simulink model "RollReducedModel_Generated"  (R2023b)
settings: Solver=FixedStepAuto  StartTime=0.0  StopTime=10.0  FixedStep=0.005  RelTol=1e-3
PreLoadFcn:
  | JointParameters
values from neighbouring files (symbols this model uses):
  B_l = 0.5    [JointParameters.m]    (also in MyDict.sldd = 0.5
                
                    
                  )
  B_u = 0.5    [JointParameters.m]    (also in MyDict.sldd = 0.5
                
                    
                  )
  FilterCoeffN = 10    [JointParameters.m]    (also in MyDict.sldd = 10.0
                
                    
                 )
  g = 9.81    [JointParameters.m]    (also in MyDict.sldd = 9.81
                
                    
                 )
  ixposkd = 0    [JointParameters.m]    (also in MyDict.sldd = 0.0
                
                    
                  )
  ixposki = 1    [JointParameters.m]    (also in MyDict.sldd = 1.0
                
                    
                  )
  ixposkp = 12    [JointParameters.m]    (also in MyDict.sldd = 12.0
                
                    
                 )
  ixvelkd = 0    [JointParameters.m]    (also in MyDict.sldd = 0.0
                
                    
                  )
  ixvelki = 5    [JointParameters.m]    (also in MyDict.sldd = 5.0
                
                    
                  )
  ixvelkp = 30    [JointParameters.m]    (also in MyDict.sldd = 30.0
                
                    
                 )
  iyposkd = 0    [JointParameters.m]    (also in MyDict.sldd = 0.0
                
                    
                  )
  iyposki = 1    [JointParameters.m]    (also in MyDict.sldd = 1.0
                
                    
                  )
  iyposkp = 10    [JointParameters.m]    (also in MyDict.sldd = 10.0
                
                    
                 )
  iyvelkd = 0    [JointParameters.m]    (also in MyDict.sldd = 0.0
                
                    
                  )
  iyvelki = 5    [JointParameters.m]    (also in MyDict.sldd = 5.0
                
                    
                  )
  iyvelkp = 20    [JointParameters.m]    (also in MyDict.sldd = 20.0
                
                    
                 )
  J_l = 0.071440709    [JointParameters.m]    (also in MyDict.sldd = 0.071440709
                
                    
          )
  J_u = 0.049103    [JointParameters.m]    (also in MyDict.sldd = 0.049103
                
                    
             )
  JointX_InitialPositionCondition = 0.27    [JointParameters.m]    (also in MyDict.sldd = 0.27
                
                    
                 )
  JointY_InitialPositionCondition = -0.33    [JointParameters.m]    (also in MyDict.sldd = -0.33
                
                    
                )
  L_cg_l = 0.102366    [JointParameters.m]    (also in MyDict.sldd = 0.102366
                
                    
             )
  L_cg_u = 0.066301    [JointParameters.m]    (also in MyDict.sldd = 0.066301
                
                    
             )
  L_l = 0.223793    [JointParameters.m]    (also in MyDict.sldd = 0.223793
                
                    
             )
  L_u = 0.227293    [JointParameters.m]    (also in MyDict.sldd = 0.227293
                
                    
             )
  mass_l = 2.495    [JointParameters.m]    (also in MyDict.sldd = 2.495
                
                    
                )
  mass_u = 2.024    [JointParameters.m]    (also in MyDict.sldd = 2.024
                
                    
                )
  PitchLowerLimit = -0.37    [JointParameters.m]    (also in MyDict.sldd = -0.37
                
                    
                )
  PitchUpperLimit = 0.27    [JointParameters.m]    (also in MyDict.sldd = 0.27
                
                    
                 )
  PitchXMotorSaturation = 50    [JointParameters.m]    (also in MyDict.sldd = 50.0
                
                    
                 )
  PitchXStartThrust = 50    [JointParameters.m]    (also in MyDict.sldd = 50.0
                
                    
                 )
  RollLowerLimit = -0.33    [JointParameters.m]    (also in MyDict.sldd = -0.33
                
                    
                )
  RollUpperLimit = 0.4    [JointParameters.m]    (also in MyDict.sldd = 0.4
                
                    
                  )
  RollYMotorSaturation = 30    [JointParameters.m]    (also in MyDict.sldd = 30.0
                
                    
                 )
  RollYStartThrust = 40    [JointParameters.m]    (also in MyDict.sldd = 40.0
                
                    
                 )
undefined symbols (not defined in the file or in its folder): DiscIntNeverNeededParam
libraries: slpidlib x4
settings Model: DataDictionary=MyDict.sldd  Creator=user  LastModifiedBy=user
settings SolverCC: AlgebraicLoopSolver=TrustRegion
settings OptimizationCC: DefaultParameterBehavior=Inlined  EnhancedBackFolding=on  PassReuseOutputArgsAs=Individual arguments  ZeroExternalMemoryAtStartup=off  ZeroInternalMemoryAtStartup=off  OptimizeBlockOrder=speed  DifferentSizesBufferReuse=on  OptimizationCustomize=off  EfficientTunableParamExpr=on
settings DebuggingCC: ParameterTunabilityLossMsg=error
settings SFSimCC: MATLABDynamicMemAlloc=off
settings RTWCC: Description=Embedded Coder  SystemTargetFile=ert.tlc  GenCodeOnly=on  TemplateMakefile=ert_default_tmf  GenerateReport=on  LaunchReport=on  DataTypeReplacement=CDataTypesFixedWidth  GenerateWebview=on  GenerateCodeMetricsReport=on
settings CodeAppCC: GenerateComments=off  IgnoreCustomStorageClasses=off  OperatorAnnotations=on  SimulinkDataObjDesc=on  SFDataObjDesc=on  SimulinkBlockComments=off
settings ERTTargetCC: TargetLangStandard=C99 (ISO)  GenerateSampleERTMain=on  SupportAbsoluteTime=off  SupportNonFinite=off  SupportComplex=off  InlinedParameterPlacement=NonHierarchical  ERTCustomFileTemplate=example_file_process.tlc  GlobalDataDefinition=InSourceFile  GlobalDataReference=InSourceFile  ERTFilePackagingFormat=Compact  MaxIdInt64=INT64_MAX  MinIdInt64=INT64_MIN  MaxIdUint64=UINT64_MAX  MaxIdInt32=INT32_MAX  MinIdInt32=INT32_MIN  MaxIdUint32=UINT32_MAX  MaxIdInt16=INT16_MAX  MinIdInt16=INT16_MIN  MaxIdUint16=UINT16_MAX  MaxIdInt8=INT8_MAX  MinIdInt8=INT8_MIN  MaxIdUint8=UINT8_MAX

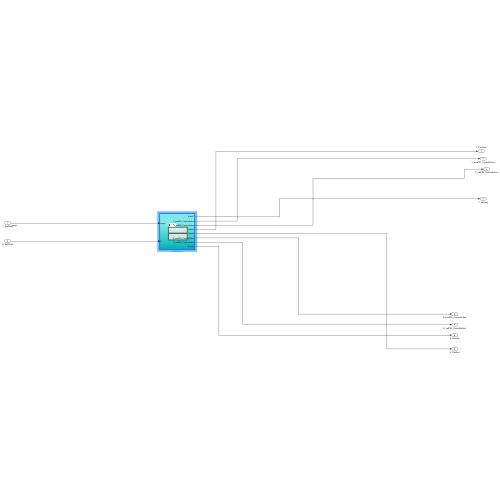
[thumbnail: Simulink's stored preview of the top-level diagram]
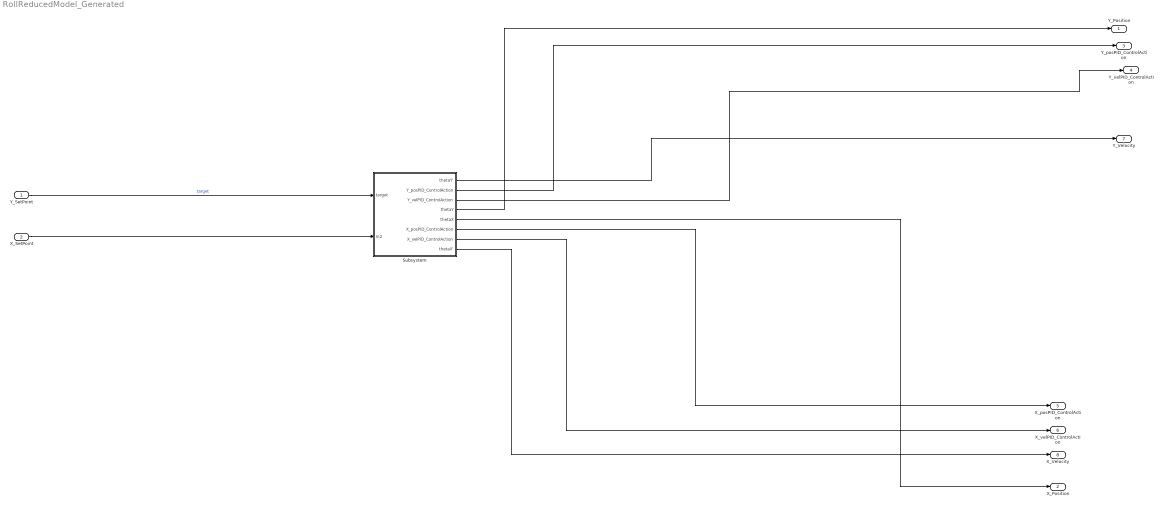
== system RollReducedModel_Generated ==
  Y_SetPoint : Inport  OutDataTypeStr=double
  X_SetPoint : Inport  Port=2  OutDataTypeStr=double
  Subsystem : Subsystem  TreatAsAtomicUnit=on
  Y_Position : Outport
  X_Position : Outport  Port=2
  Y_posPID_ControlAction : Outport  Port=3
  Y_velPID_ControlAction : Outport  Port=4
  X_posPID_ControlAction : Outport  Port=5
  X_velPID_ControlAction : Outport  Port=6
  Y_Velocity : Outport  Port=7
  X_Velocity : Outport  Port=8
  wires:
  Y_SetPoint/1 -> Subsystem/1(target)  "target"
  X_SetPoint/1 -> Subsystem/2(In2)
  Subsystem/1(thetaY') -> Y_Velocity/1
  Subsystem/2(Y_posPID_ControlAction) -> Y_posPID_ControlAction/1
  Subsystem/3(Y_velPID_ControlAction) -> Y_velPID_ControlAction/1
  Subsystem/4(thetaY) -> Y_Position/1
  Subsystem/5(thetaX) -> X_Position/1
  Subsystem/6(X_posPID_ControlAction) -> X_posPID_ControlAction/1
  Subsystem/7(X_velPID_ControlAction) -> X_velPID_ControlAction/1
  Subsystem/8(thetaX') -> X_Velocity/1

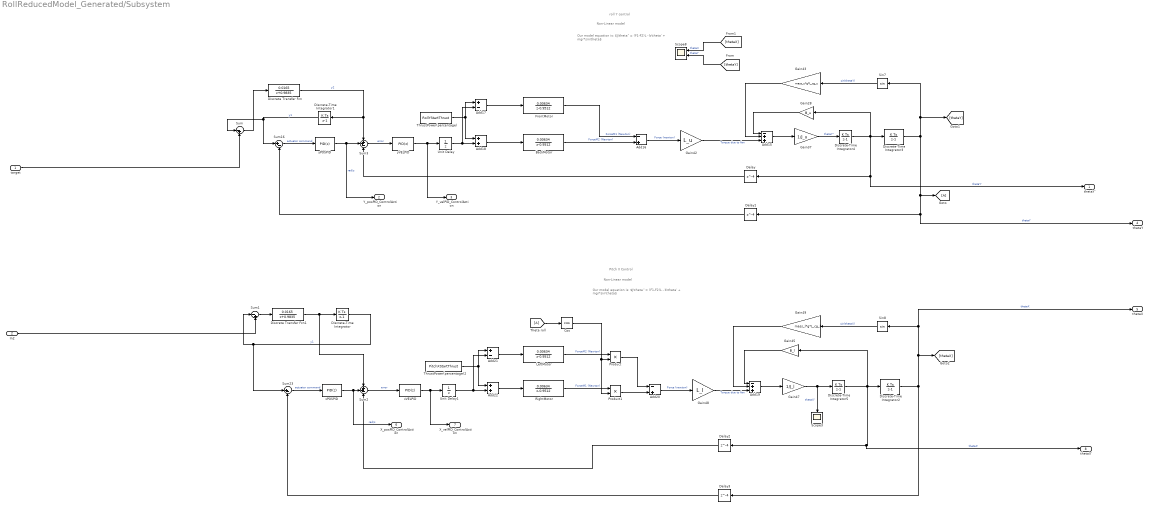
== system RollReducedModel_Generated/Subsystem ==
  note: Our model equation is:
      | $J\theta'' = (F1-F2)L - b\theta' + mgr*sin\theta$
  note: Our model equation is:
      | $J\theta'' = (F1-F2)L - b\theta' + mgr*sin\theta$
  note: Non-Linear model
  note: Pitch X Control
  note: Non-Linear model
  note: roll Y control
  target : Inport
  In2 : Inport  Port=2
  Add15 : Sum  Inputs=-++
  Add16 : Sum  Inputs=-+
  Add17 : Sum  Inputs=+-
  Add18 : Sum
  Add19 : Sum  Inputs=-++
  Add20 : Sum  Inputs=-+
  Add21 : Sum  Inputs=+-
  Add22 : Sum
  BackMotor : DiscreteTransferFcn  Numerator=[0.00634]  Denominator=[1 -0.9512]
  Cos : Trigonometry  Operator=cos
  Delay{,1..3} (4 alike) : Delay  DelayLength=4
  Discrete Transfer Fcn : DiscreteTransferFcn  Numerator=[0.0165]  Denominator=[1 0.9835]
  Discrete Transfer Fcn1 : DiscreteTransferFcn  Numerator=[0.0165]  Denominator=[1 0.9835]
  Discrete-Time Integrator{,1,4..5} (4 alike) : DiscreteIntegrator  SampleTime=-1  ICPrevOutput=DiscIntNeverNeededParam  ICPrevScaledInput=DiscIntNeverNeededParam
  Discrete-Time Integrator2 : DiscreteIntegrator  InitialCondition=JointX_InitialPositionCondition  SampleTime=-1  LimitOutput=on  UpperSaturationLimit=PitchUpperLimit  LowerSaturationLimit=PitchLowerLimit  ICPrevOutput=DiscIntNeverNeededParam  ICPrevScaledInput=DiscIntNeverNeededParam
  Discrete-Time Integrator3 : DiscreteIntegrator  InitialCondition=JointY_InitialPositionCondition  SampleTime=-1  LimitOutput=on  UpperSaturationLimit=RollUpperLimit  LowerSaturationLimit=RollLowerLimit  ICPrevOutput=DiscIntNeverNeededParam  ICPrevScaledInput=DiscIntNeverNeededParam
  FrontMotor : DiscreteTransferFcn  Numerator=[0.00634]  Denominator=[1 -0.9512]
  Gain28 : Gain  Gain=B_u
  Gain37 : Gain  Gain=1/J_u
  Gain42 : Gain  Gain=L_u
  Gain43 : Gain  Gain=mass_u*g*L_cg_u
  Gain45 : Gain  Gain=B_l
  Gain47 : Gain  Gain=1/J_l
  Gain48 : Gain  Gain=L_l
  Gain49 : Gain  Gain=mass_l*g*L_cg_l
  Goto : Goto
  LeftMotor : DiscreteTransferFcn  Numerator=[0.00634]  Denominator=[1 -0.9512]
  Product : Product
  Product1 : Product
  RightMotor : DiscreteTransferFcn  Numerator=[0.00634]  Denominator=[1 -0.9512]
  Scope3 : Scope
  Scope8 : Scope  NumInputPorts=2
  Sin7 : Trigonometry
  Sin8 : Trigonometry
  Sum : Sum  Inputs=|-+
  Sum1 : Sum  Inputs=|-+
  Sum16 : Sum  Inputs=|+-
  Sum2 : Sum  Inputs=++-
  Sum23 : Sum  Inputs=|+-
  Sum3 : Sum  Inputs=++-
  Theta roll : From
  ThrustPower(percentage) : Constant  Value=RollYStartThrust
  ThrustPower(percentage)2 : Constant  Value=PitchXStartThrust
  Unit Delay : UnitDelay  SampleTime=-1  HasFrameUpgradeWarning=on
  Unit Delay1 : UnitDelay  SampleTime=-1  HasFrameUpgradeWarning=on
  xPOSPID : slpidlib/PID Controller  Controller=PID  Form=Parallel  TimeDomain=Discrete-time  UseExternalTs=off  SampleTime=0.005  IntegratorMethod=Forward Euler  FilterMethod=Forward Euler  ControllerParametersSource=internal  P=ixposkp  I=ixposki  UseKiTs=off  D=ixposkd  N=FilterCoeffN  UseFilter=on  TunerSelectOption=Transfer Function Based (PID Tuner App)  InitialConditionSource=internal  InitialConditionForIntegrator=0  InitialConditionForFilter=0  DifferentiatorICPrevScaledInput=0  ExternalReset=none  TrackingMode=off  Kt=1  LimitOutput=on  SatLimitsSource=internal  UpperSaturationLimit=1  LowerSaturationLimit=-1  LinearizeAsGain=on  AntiWindupMode=clamping  Kb=1  LimitIntegrator=off  UpperIntegratorSaturationLimit=inf  LowerIntegratorSaturationLimit=-inf  POutMin=[]  POutMax=[]  IOutMin=[]  IOutMax=[]  DOutMin=[]  DOutMax=[]  NOutMin=[]  NOutMax=[]  SumOutMin=[]  SumOutMax=[]  SaturationOutMin=[]  SaturationOutMax=[]  PParamMin=[]  PParamMax=[]  IParamMin=[]  IParamMax=[]  DParamMin=[]  DParamMax=[]  NParamMin=[]  NParamMax=[]  KbParamMin=[]  KbParamMax=[]  KtParamMin=[]  KtParamMax=[]  KbOutMin=[]  KbOutMax=[]  KtOutMin=[]  KtOutMax=[]  IntegratorOutMin=[]  IntegratorOutMax=[]  FilterOutMin=[]  FilterOutMax=[]  SumI1OutMin=[]  SumI1OutMax=[]  SumI2OutMin=[]  SumI2OutMax=[]  SumI3OutMin=[]  SumI3OutMax=[]  SumI4OutMin=[]  SumI4OutMax=[]  SumDOutMin=[]  SumDOutMax=[]  DifferentiatorOutMin=[]  DifferentiatorOutMax=[]  FilterDiffOutCoefMin=[]  FilterDiffOutCoefMax=[]  ReciprocalOutMin=[]  ReciprocalOutMax=[]  SumDenOutMin=[]  SumDenOutMax=[]  SumNumOutMin=[]  SumNumOutMax=[]  DivideOutMin=[]  DivideOutMax=[]  UdiffTsProdOutMin=[]  UdiffTsProdOutMax=[]  NTsProdOutMin=[]  NTsProdOutMax=[]  UintegralTsProdOutMin=[]  UintegralTsProdOutMax=[]  UngainTsProdOutMin=[]  UngainTsProdOutMax=[]  ClampingZeroOutDataTypeStr=Inherit: Inherit via back propagation  ClampingZeroOutMin=[]  ClampingZeroOutMax=[]  FilterDenConstantOutDataTypeStr=Inherit: Inherit via back propagation  FilterDenConstantOutMin=[]  FilterDenConstantOutMax=[]  PCopyOutDataTypeStr=Inherit: Inherit via back propagation  PCopyOutMin=[]  PCopyOutMax=[]  NCopyOutDataTypeStr=Inherit: Inherit via back propagation  NCopyOutMin=[]  NCopyOutMax=[]  IntegratorContinuousStateAttributes=''  IntegratorStateMustResolveToSignalObject=off  IntegratorRTWStateStorageClass=Auto  FilterContinuousStateAttributes=''  FilterStateMustResolveToSignalObject=off  FilterRTWStateStorageClass=Auto  ParallelPVariant=InternalParameters  IdealPVariant=Disabled  IVariant=InternalParameters  DVariant=InternalParameters  IntegratorVariant=Discrete  SatVariant=Enabled  AWVariant=DiscClampingParallel  PCopyVariant=Disabled  TRVariant=Disabled  FdbkBlocksVariant=Forward  IdealPFdbkVariant=Disabled  SatFdbkVariant=Disabled  DerivativeFilterVariant=ForwardEulerFilter  NVariant=InternalParameters  NCopyVariant=Disabled  FilterICVariant=InternalICsFilter  IntegratorICVariant=InternalICs  ExternalResetVariant=Disabled  TRSumVariant=Passthrough  SumFdbkVariant=Disabled  SumVariant=Sum_PID  TsampFilterVariant=InternalTs  TsampNgainVariant=Passthrough  TsampIntegralVariant=Disabled_SignalSpec  ExternalSaturationOutDataTypeStr=Inherit: Same as second input
  xVELPID : slpidlib/PID Controller  Controller=PID  Form=Parallel  TimeDomain=Discrete-time  UseExternalTs=off  SampleTime=0.005  IntegratorMethod=Forward Euler  FilterMethod=Forward Euler  ControllerParametersSource=internal  P=ixvelkp*0.4  I=ixvelki*0.4  UseKiTs=off  D=ixvelkd  N=FilterCoeffN  UseFilter=on  TunerSelectOption=Transfer Function Based (PID Tuner App)  InitialConditionSource=internal  InitialConditionForIntegrator=0  InitialConditionForFilter=0  DifferentiatorICPrevScaledInput=0  ExternalReset=none  TrackingMode=off  Kt=1  LimitOutput=on  SatLimitsSource=internal  UpperSaturationLimit=PitchXMotorSaturation  LowerSaturationLimit=-PitchXMotorSaturation  LinearizeAsGain=on  AntiWindupMode=clamping  Kb=1  LimitIntegrator=off  UpperIntegratorSaturationLimit=inf  LowerIntegratorSaturationLimit=-inf  POutMin=[]  POutMax=[]  IOutMin=[]  IOutMax=[]  DOutMin=[]  DOutMax=[]  NOutMin=[]  NOutMax=[]  SumOutMin=[]  SumOutMax=[]  SaturationOutMin=[]  SaturationOutMax=[]  PParamMin=[]  PParamMax=[]  IParamMin=[]  IParamMax=[]  DParamMin=[]  DParamMax=[]  NParamMin=[]  NParamMax=[]  KbParamMin=[]  KbParamMax=[]  KtParamMin=[]  KtParamMax=[]  KbOutMin=[]  KbOutMax=[]  KtOutMin=[]  KtOutMax=[]  IntegratorOutMin=[]  IntegratorOutMax=[]  FilterOutMin=[]  FilterOutMax=[]  SumI1OutMin=[]  SumI1OutMax=[]  SumI2OutMin=[]  SumI2OutMax=[]  SumI3OutMin=[]  SumI3OutMax=[]  SumI4OutMin=[]  SumI4OutMax=[]  SumDOutMin=[]  SumDOutMax=[]  DifferentiatorOutMin=[]  DifferentiatorOutMax=[]  FilterDiffOutCoefMin=[]  FilterDiffOutCoefMax=[]  ReciprocalOutMin=[]  ReciprocalOutMax=[]  SumDenOutMin=[]  SumDenOutMax=[]  SumNumOutMin=[]  SumNumOutMax=[]  DivideOutMin=[]  DivideOutMax=[]  UdiffTsProdOutMin=[]  UdiffTsProdOutMax=[]  NTsProdOutMin=[]  NTsProdOutMax=[]  UintegralTsProdOutMin=[]  UintegralTsProdOutMax=[]  UngainTsProdOutMin=[]  UngainTsProdOutMax=[]  ClampingZeroOutDataTypeStr=Inherit: Inherit via back propagation  ClampingZeroOutMin=[]  ClampingZeroOutMax=[]  FilterDenConstantOutDataTypeStr=Inherit: Inherit via back propagation  FilterDenConstantOutMin=[]  FilterDenConstantOutMax=[]  PCopyOutDataTypeStr=Inherit: Inherit via back propagation  PCopyOutMin=[]  PCopyOutMax=[]  NCopyOutDataTypeStr=Inherit: Inherit via back propagation  NCopyOutMin=[]  NCopyOutMax=[]  IntegratorContinuousStateAttributes=''  IntegratorStateMustResolveToSignalObject=off  IntegratorRTWStateStorageClass=Auto  FilterContinuousStateAttributes=''  FilterStateMustResolveToSignalObject=off  FilterRTWStateStorageClass=Auto  ParallelPVariant=InternalParameters  IdealPVariant=Disabled  IVariant=InternalParameters  DVariant=InternalParameters  IntegratorVariant=Discrete  SatVariant=Enabled  AWVariant=DiscClampingParallel  PCopyVariant=Disabled  TRVariant=Disabled  FdbkBlocksVariant=Forward  IdealPFdbkVariant=Disabled  SatFdbkVariant=Disabled  DerivativeFilterVariant=ForwardEulerFilter  NVariant=InternalParameters  NCopyVariant=Disabled  FilterICVariant=InternalICsFilter  IntegratorICVariant=InternalICs  ExternalResetVariant=Disabled  TRSumVariant=Passthrough  SumFdbkVariant=Disabled  SumVariant=Sum_PID  TsampFilterVariant=InternalTs  TsampNgainVariant=Passthrough  TsampIntegralVariant=Disabled_SignalSpec  ExternalSaturationOutDataTypeStr=Inherit: Same as second input
  yPOSPID : slpidlib/PID Controller  Controller=PID  Form=Parallel  TimeDomain=Discrete-time  UseExternalTs=off  SampleTime=0.005  IntegratorMethod=Forward Euler  FilterMethod=Forward Euler  ControllerParametersSource=internal  P=iyposkp  I=iyposki  UseKiTs=off  D=iyposkd  N=FilterCoeffN  UseFilter=on  TunerSelectOption=Transfer Function Based (PID Tuner App)  InitialConditionSource=internal  InitialConditionForIntegrator=0  InitialConditionForFilter=0  DifferentiatorICPrevScaledInput=0  ExternalReset=none  TrackingMode=off  Kt=1  LimitOutput=on  SatLimitsSource=internal  UpperSaturationLimit=1  LowerSaturationLimit=-1  LinearizeAsGain=on  AntiWindupMode=clamping  Kb=1  LimitIntegrator=off  UpperIntegratorSaturationLimit=inf  LowerIntegratorSaturationLimit=-inf  POutMin=[]  POutMax=[]  IOutMin=[]  IOutMax=[]  DOutMin=[]  DOutMax=[]  NOutMin=[]  NOutMax=[]  SumOutMin=[]  SumOutMax=[]  SaturationOutMin=[]  SaturationOutMax=[]  PParamMin=[]  PParamMax=[]  IParamMin=[]  IParamMax=[]  DParamMin=[]  DParamMax=[]  NParamMin=[]  NParamMax=[]  KbParamMin=[]  KbParamMax=[]  KtParamMin=[]  KtParamMax=[]  KbOutMin=[]  KbOutMax=[]  KtOutMin=[]  KtOutMax=[]  IntegratorOutMin=[]  IntegratorOutMax=[]  FilterOutMin=[]  FilterOutMax=[]  SumI1OutMin=[]  SumI1OutMax=[]  SumI2OutMin=[]  SumI2OutMax=[]  SumI3OutMin=[]  SumI3OutMax=[]  SumI4OutMin=[]  SumI4OutMax=[]  SumDOutMin=[]  SumDOutMax=[]  DifferentiatorOutMin=[]  DifferentiatorOutMax=[]  FilterDiffOutCoefMin=[]  FilterDiffOutCoefMax=[]  ReciprocalOutMin=[]  ReciprocalOutMax=[]  SumDenOutMin=[]  SumDenOutMax=[]  SumNumOutMin=[]  SumNumOutMax=[]  DivideOutMin=[]  DivideOutMax=[]  UdiffTsProdOutMin=[]  UdiffTsProdOutMax=[]  NTsProdOutMin=[]  NTsProdOutMax=[]  UintegralTsProdOutMin=[]  UintegralTsProdOutMax=[]  UngainTsProdOutMin=[]  UngainTsProdOutMax=[]  ClampingZeroOutDataTypeStr=Inherit: Inherit via back propagation  ClampingZeroOutMin=[]  ClampingZeroOutMax=[]  FilterDenConstantOutDataTypeStr=Inherit: Inherit via back propagation  FilterDenConstantOutMin=[]  FilterDenConstantOutMax=[]  PCopyOutDataTypeStr=Inherit: Inherit via back propagation  PCopyOutMin=[]  PCopyOutMax=[]  NCopyOutDataTypeStr=Inherit: Inherit via back propagation  NCopyOutMin=[]  NCopyOutMax=[]  IntegratorContinuousStateAttributes=''  IntegratorStateMustResolveToSignalObject=off  IntegratorRTWStateStorageClass=Auto  FilterContinuousStateAttributes=''  FilterStateMustResolveToSignalObject=off  FilterRTWStateStorageClass=Auto  ParallelPVariant=InternalParameters  IdealPVariant=Disabled  IVariant=InternalParameters  DVariant=InternalParameters  IntegratorVariant=Discrete  SatVariant=Enabled  AWVariant=DiscClampingParallel  PCopyVariant=Disabled  TRVariant=Disabled  FdbkBlocksVariant=Forward  IdealPFdbkVariant=Disabled  SatFdbkVariant=Disabled  DerivativeFilterVariant=ForwardEulerFilter  NVariant=InternalParameters  NCopyVariant=Disabled  FilterICVariant=InternalICsFilter  IntegratorICVariant=InternalICs  ExternalResetVariant=Disabled  TRSumVariant=Passthrough  SumFdbkVariant=Disabled  SumVariant=Sum_PID  TsampFilterVariant=InternalTs  TsampNgainVariant=Passthrough  TsampIntegralVariant=Disabled_SignalSpec  ExternalSaturationOutDataTypeStr=Inherit: Same as second input
  yVELPID : slpidlib/PID Controller  Controller=PID  Form=Parallel  TimeDomain=Discrete-time  UseExternalTs=off  SampleTime=0.005  IntegratorMethod=Forward Euler  FilterMethod=Forward Euler  ControllerParametersSource=internal  P=iyvelkp  I=iyvelki  UseKiTs=off  D=iyvelkd  N=FilterCoeffN  UseFilter=on  TunerSelectOption=Transfer Function Based (PID Tuner App)  InitialConditionSource=internal  InitialConditionForIntegrator=0  InitialConditionForFilter=0  DifferentiatorICPrevScaledInput=0  ExternalReset=none  TrackingMode=off  Kt=1  LimitOutput=on  SatLimitsSource=internal  UpperSaturationLimit=RollYMotorSaturation  LowerSaturationLimit=-RollYMotorSaturation  LinearizeAsGain=on  AntiWindupMode=clamping  Kb=1  LimitIntegrator=off  UpperIntegratorSaturationLimit=inf  LowerIntegratorSaturationLimit=-inf  POutMin=[]  POutMax=[]  IOutMin=[]  IOutMax=[]  DOutMin=[]  DOutMax=[]  NOutMin=[]  NOutMax=[]  SumOutMin=[]  SumOutMax=[]  SaturationOutMin=[]  SaturationOutMax=[]  PParamMin=[]  PParamMax=[]  IParamMin=[]  IParamMax=[]  DParamMin=[]  DParamMax=[]  NParamMin=[]  NParamMax=[]  KbParamMin=[]  KbParamMax=[]  KtParamMin=[]  KtParamMax=[]  KbOutMin=[]  KbOutMax=[]  KtOutMin=[]  KtOutMax=[]  IntegratorOutMin=[]  IntegratorOutMax=[]  FilterOutMin=[]  FilterOutMax=[]  SumI1OutMin=[]  SumI1OutMax=[]  SumI2OutMin=[]  SumI2OutMax=[]  SumI3OutMin=[]  SumI3OutMax=[]  SumI4OutMin=[]  SumI4OutMax=[]  SumDOutMin=[]  SumDOutMax=[]  DifferentiatorOutMin=[]  DifferentiatorOutMax=[]  FilterDiffOutCoefMin=[]  FilterDiffOutCoefMax=[]  ReciprocalOutMin=[]  ReciprocalOutMax=[]  SumDenOutMin=[]  SumDenOutMax=[]  SumNumOutMin=[]  SumNumOutMax=[]  DivideOutMin=[]  DivideOutMax=[]  UdiffTsProdOutMin=[]  UdiffTsProdOutMax=[]  NTsProdOutMin=[]  NTsProdOutMax=[]  UintegralTsProdOutMin=[]  UintegralTsProdOutMax=[]  UngainTsProdOutMin=[]  UngainTsProdOutMax=[]  ClampingZeroOutDataTypeStr=Inherit: Inherit via back propagation  ClampingZeroOutMin=[]  ClampingZeroOutMax=[]  FilterDenConstantOutDataTypeStr=Inherit: Inherit via back propagation  FilterDenConstantOutMin=[]  FilterDenConstantOutMax=[]  PCopyOutDataTypeStr=Inherit: Inherit via back propagation  PCopyOutMin=[]  PCopyOutMax=[]  NCopyOutDataTypeStr=Inherit: Inherit via back propagation  NCopyOutMin=[]  NCopyOutMax=[]  IntegratorContinuousStateAttributes=''  IntegratorStateMustResolveToSignalObject=off  IntegratorRTWStateStorageClass=Auto  FilterContinuousStateAttributes=''  FilterStateMustResolveToSignalObject=off  FilterRTWStateStorageClass=Auto  ParallelPVariant=InternalParameters  IdealPVariant=Disabled  IVariant=InternalParameters  DVariant=InternalParameters  IntegratorVariant=Discrete  SatVariant=Enabled  AWVariant=DiscClampingParallel  PCopyVariant=Disabled  TRVariant=Disabled  FdbkBlocksVariant=Forward  IdealPFdbkVariant=Disabled  SatFdbkVariant=Disabled  DerivativeFilterVariant=ForwardEulerFilter  NVariant=InternalParameters  NCopyVariant=Disabled  FilterICVariant=InternalICsFilter  IntegratorICVariant=InternalICs  ExternalResetVariant=Disabled  TRSumVariant=Passthrough  SumFdbkVariant=Disabled  SumVariant=Sum_PID  TsampFilterVariant=InternalTs  TsampNgainVariant=Passthrough  TsampIntegralVariant=Disabled_SignalSpec  ExternalSaturationOutDataTypeStr=Inherit: Same as second input
  thetaY' : Outport
  Y_posPID_ControlAction : Outport  Port=2
  Y_velPID_ControlAction : Outport  Port=3
  thetaY : Outport  Port=4
  thetaX : Outport  Port=5
  X_posPID_ControlAction : Outport  Port=6
  X_velPID_ControlAction : Outport  Port=7
  thetaX' : Outport  Port=8
  wires:
  Discrete-Time Integrator5/1 -> Discrete-Time Integrator2/1, thetaX'/1, Delay2/1, Gain45/1  "thetaX'"
  xPOSPID/1 -> X_posPID_ControlAction/1, Sum2/2  "rad/s"
  Discrete-Time Integrator3/1 -> thetaY/1, Delay1/1, Goto/1, Sin7/1, [thetaY]  "thetaY"
  Discrete-Time Integrator1/1 -> Sum/1, Sum16/1  "y1"
  Delay1/1 -> Sum16/2
  Sin8/1 -> Gain49/1  "sin(thetaX)"
  Discrete Transfer Fcn/1 -> Sum3/1, Discrete-Time Integrator1/1  "y2"
  Theta roll/1 -> Cos/1
  Discrete-Time Integrator/1 -> Sum23/1, Sum1/1  "y1"
  Gain48/1 -> Add19/3  "Torque due to fan"
  [thetaY] -> Scope8/2  "thetaY"
  Sum23/1 -> xPOSPID/1  "actuator command"
  Sum16/1 -> yPOSPID/1  "actuator command"
  Add15/1 -> Gain37/1
  Discrete Transfer Fcn1/1 -> Discrete-Time Integrator/1, Sum2/1
  Unit Delay1/1 -> Add22/2, Add21/2
  Gain45/1 -> Add19/1
  Add16/1 -> Gain42/1  "Force (newton)"
  Cos/1 -> Product1/2, Product/2
  Discrete-Time Integrator2/1 -> Delay3/1, thetaX/1, Sin8/1, [thetaX]  "thetaX"
  FrontMotor/1 -> Add16/1  "ForceM1 (Newton)"
  Add20/1 -> Gain48/1  "Force (newton)"
  ThrustPower(percentage)2/1 -> Add22/1, Add21/1
  xVELPID/1 -> X_velPID_ControlAction/1, Unit Delay1/1
  Add19/1 -> Gain47/1
  Gain49/1 -> Add19/2
  Delay2/1 -> Sum2/3
  Gain47/1 -> Discrete-Time Integrator5/1, Scope3/1  "thetaX''"
  Gain28/1 -> Add15/1
  Sum/1 -> Discrete Transfer Fcn/1
  Product1/1 -> Add20/2
  Unit Delay/1 -> Add17/2, Add18/2
  yPOSPID/1 -> Y_posPID_ControlAction/1, Sum3/2  "rad/s"
  BackMotor/1 -> Add16/2  "ForceM2 (Newton)"
  [thetaX] -> Scope8/1  "thetaX"
  Discrete-Time Integrator4/1 -> Discrete-Time Integrator3/1, thetaY'/1, Delay/1, Gain28/1  "thetaY'"
  Sum2/1 -> xVELPID/1  "error"
  Gain42/1 -> Add15/3  "Torque due to fan"
  Product/1 -> Add20/1
  Sin7/1 -> Gain43/1  "sin(thetaY)"
  target/1 -> Sum/2
  Sum3/1 -> yVELPID/1  "error"
  ThrustPower(percentage)/1 -> Add18/1, Add17/1
  yVELPID/1 -> Y_velPID_ControlAction/1, Unit Delay/1
  Gain43/1 -> Add15/2
  Delay/1 -> Sum3/3
  Add17/1 -> FrontMotor/1
  Sum1/1 -> Discrete Transfer Fcn1/1
  Delay3/1 -> Sum23/2
  Add21/1 -> LeftMotor/1
  LeftMotor/1 -> Product/1  "ForceM2 (Newton)"
  Add18/1 -> BackMotor/1
  Gain37/1 -> Discrete-Time Integrator4/1  "thetaY''"
  Add22/1 -> RightMotor/1
  RightMotor/1 -> Product1/1  "ForceM1 (Newton)"
  In2/1 -> Sum1/2
